simulink model "online_multi_sim_control"  (R2019b)
settings: Solver=FixedStepAuto  StartTime=0.0  StopTime=30  RelTol=1e-3
settings Model: Creator=sanim  LastModifiedBy=Dell
settings DataIOCC: ReturnWorkspaceOutputs=off
settings DebuggingCC: ArithmeticOperatorsInVariantConditions=warning
settings SFSimCC: CustomCodeUndefinedFunction=UseInterfaceOnly

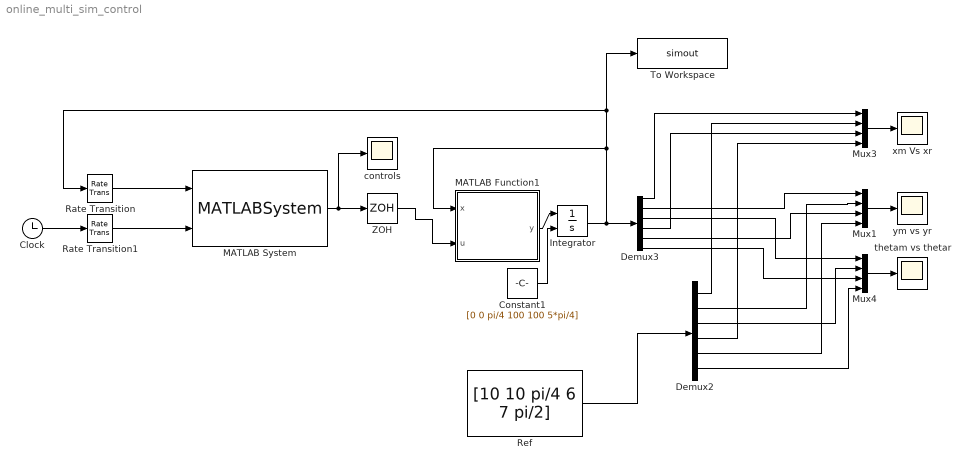
== system online_multi_sim_control ==
  Clock : Clock
  Constant1 : Constant  Value=[0 0 pi/4 100 100 5*pi/4]
  Demux2 : Demux  Outputs=6
  Demux3 : Demux  Outputs=6
  Integrator : Integrator  InitialConditionSource=external  InitialCondition=[1 0]'
  MATLAB Function1 : MATLAB Function  TreatAsAtomicUnit=on
  MATLAB System : MATLABSystem  System=multidistance  SimulateUsing=Interpreted execution
      mask Type: multidistance
      mask Display:
      | disp('multidistance');
      | port_label('input',1,'x');
      | port_label('input',2,'t');
      | port_label('output',1,'u');
  Mux1 : Mux
  Mux3 : Mux
  Mux4 : Mux
  Rate Transition : RateTransition  OutPortSampleTime=0.1
  Rate Transition1 : RateTransition  OutPortSampleTime=0.1
  Ref : Constant  Value=[10 10 pi/4 6 7 pi/2]  VectorParams1D=off
  To Workspace : ToWorkspace  VariableName=simout  SaveFormat=Timeseries  SampleTime=-1
  ZOH : ZeroOrderHold  SampleTime=0.5
  controls : Scope
  thetam vs thetar : Scope
  xm Vs xr : Scope
  ym vs yr : Scope
  wires:
  Ref/1 -> Demux2/1
  Rate Transition/1 -> MATLAB System/1
  MATLAB System/1 -> controls/1, ZOH/1
  Integrator/1 -> To Workspace/1, Rate Transition/1, MATLAB Function1/1(x), Demux3/1
  Rate Transition1/1 -> MATLAB System/2
  ZOH/1 -> MATLAB Function1/2(u)
  Clock/1 -> Rate Transition1/1
  Mux3/1 -> xm Vs xr/1
  Mux1/1 -> ym vs yr/1
  Mux4/1 -> thetam vs thetar/1
  MATLAB Function1/1(y) -> Integrator/1
  Constant1/1 -> Integrator/2
  Demux3/1 -> Mux3/1
  Demux3/2 -> Mux1/1
  Demux3/3 -> Mux4/1
  Demux3/4 -> Mux3/3
  Demux3/5 -> Mux1/3
  Demux3/6 -> Mux4/3
  Demux2/1 -> Mux3/2
  Demux2/2 -> Mux1/2
  Demux2/3 -> Mux4/2
  Demux2/4 -> Mux3/4
  Demux2/5 -> Mux1/4
  Demux2/6 -> Mux4/4

== matlab function online_multi_sim_control/MATLAB Function1 ==
  data: x input; y output; u input
function y = rhs(x,u)
%#codegen
% 
 y=[(u(1)*cos(x(3)));(u(1)*sin(x(3)));u(2);(u(3)*cos(x(6)));(u(3)*sin(x(6)));u(4)];


end
